simulink model "TestPerturacionesReferencia"  (R2018b)
settings: Solver=VariableStepAuto  StartTime=0.0  StopTime=40  RelTol=1e-3
libraries: cstblocks x4
settings Model: Creator=JUAN DAVID  LastModifiedBy=JUAN DAVID

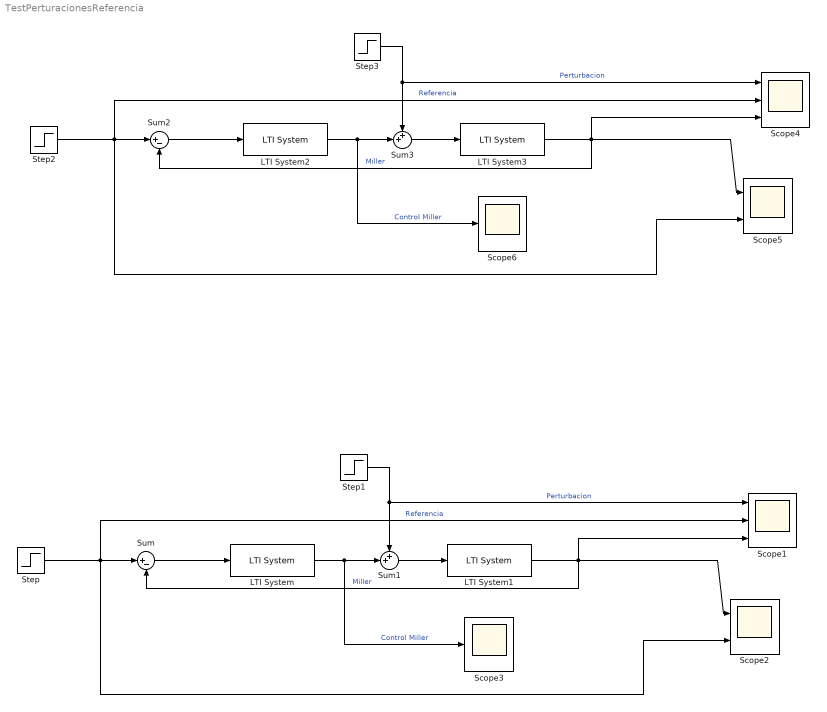
== system TestPerturacionesReferencia ==
  LTI System : cstblocks/LTI System  sys=Gs  IC=[]
  LTI System1 : cstblocks/LTI System  sys=C8  IC=[]
  LTI System2 : cstblocks/LTI System  sys=Gs  IC=[]
  LTI System3 : cstblocks/LTI System  sys=C8  IC=[]
  Scope1 : Scope  NumInputPorts=3
  Scope2 : Scope  NumInputPorts=2
  Scope3 : Scope
  Scope4 : Scope  NumInputPorts=3
  Scope5 : Scope  NumInputPorts=2
  Scope6 : Scope
  Step : Step  SampleTime=0
  Step1 : Step  Time=5  After=0.5  SampleTime=0
  Step2 : Step  SampleTime=0
  Step3 : Step  Time=5  After=0.5  SampleTime=0
  Sum : Sum  Inputs=|+-
  Sum1 : Sum  Inputs=++|
  Sum2 : Sum  Inputs=|+-
  Sum3 : Sum  Inputs=++|
  wires:
  LTI System/1 -> Scope3/1, Sum1/2  "Control Miller"
  Sum1/1 -> LTI System1/1
  Sum/1 -> LTI System/1
  Step/1 -> Scope1/2, Sum/1, Scope2/2  "Referencia"
  LTI System1/1 -> Scope1/3, Sum/2, Scope2/1  "Miller"
  Step1/1 -> Scope1/1, Sum1/1  "Perturbacion"
  LTI System3/1 -> Scope4/3, Sum2/2, Scope5/1  "Miller"
  Step3/1 -> Scope4/1, Sum3/1  "Perturbacion"
  Step2/1 -> Scope4/2, Sum2/1, Scope5/2  "Referencia"
  LTI System2/1 -> Scope6/1, Sum3/2  "Control Miller"
  Sum3/1 -> LTI System3/1
  Sum2/1 -> LTI System2/1
